simulink model "InvertedPendulum_DLQG_Simulink2020b"  (R2021b)
settings: Solver=ode4  StartTime=0.0  StopTime=SIM_TIME  FixedStep=STEP_SIZE  RelTol=1e-3
undefined symbols (not defined in the file): b, c, C_KF, F_KF, g, G_KF, I, K_opt, l, L_KF, m, M, N, theta0, theta_dot0, Ts, V2d, x0, x0_hat, x_dot0, x_ref0, yss
settings Model: Creator=roga  LastModifiedBy=roga
settings SolverCC: AlgebraicLoopSolver=TrustRegion
settings DataIOCC: ReturnWorkspaceOutputs=off
settings DebuggingCC: SFMachineParentedDataDiag=warning

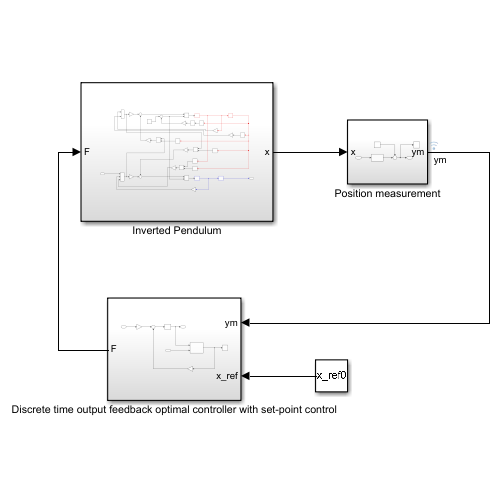
[thumbnail: Simulink's stored preview of the top-level diagram]
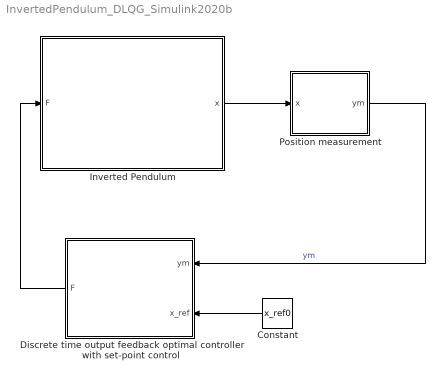
== system InvertedPendulum_DLQG_Simulink2020b ==
  Constant : Constant  Value=x_ref0  SampleTime=Ts
  Discrete time output feedback optimal controller with set-point control : Subsystem
  Inverted Pendulum : Subsystem
  Position measurement : Subsystem
  wires:
  Discrete time output feedback optimal controller with set-point control/1(F) -> Inverted Pendulum/1(F)
  Inverted Pendulum/1(x) -> Position measurement/1(x)
  Position measurement/1(ym) -> Discrete time output feedback optimal controller with set-point control/1(ym)  "ym"
  Constant/1 -> Discrete time output feedback optimal controller with set-point control/2(x_ref)

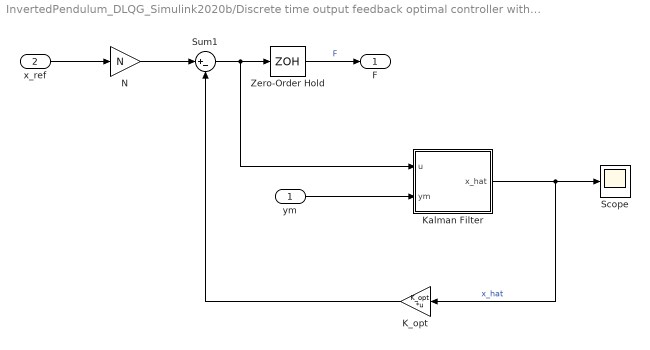
== system InvertedPendulum_DLQG_Simulink2020b/Discrete time output feedback optimal controller with set-point control ==
  ym : Inport
  x_ref : Inport  Port=2
  K_opt : Gain  Gain=K_opt  Multiplication=Matrix(K*u) (u vector)
  Kalman Filter : Subsystem
  N : Gain  Gain=N
  Scope : Scope
  Sum1 : Sum  Inputs=|+-
  Zero-Order Hold : ZeroOrderHold  SampleTime=Ts
  F : Outport
  wires:
  K_opt/1 -> Sum1/2
  Sum1/1 -> Kalman Filter/1(u), Zero-Order Hold/1
  Zero-Order Hold/1 -> F/1  "F"
  ym/1 -> Kalman Filter/2(ym)
  Kalman Filter/1(x_hat) -> Scope/1, K_opt/1  "x_hat"
  x_ref/1 -> N/1
  N/1 -> Sum1/1

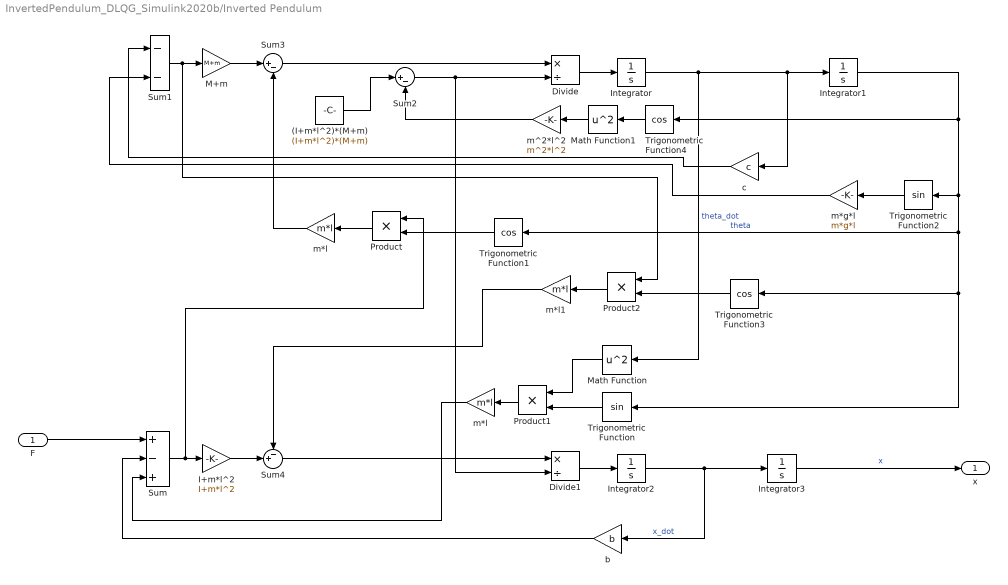
== system InvertedPendulum_DLQG_Simulink2020b/Inverted Pendulum ==
  F : Inport
  (I+m*l^2)*(M+m) : Constant  Value=(I+m*l^2)*(M+m)
  Divide : Product  Inputs=*/
  Divide1 : Product  Inputs=*/
  I+m*l^2 : Gain  Gain=I+m*l^2
  Integrator : Integrator  Priority=1  InitialCondition=theta_dot0  ContinuousStateAttributes='pendulum.angular.velocity'
  Integrator1 : Integrator  Priority=2  InitialCondition=theta0  UpperSaturationLimit=pi  LowerSaturationLimit=-pi  ContinuousStateAttributes='pendulum.angular.position'
  Integrator2 : Integrator  Priority=3  InitialCondition=x_dot0  ContinuousStateAttributes='trolley.horizontal.velocity'
  Integrator3 : Integrator  Priority=4  InitialCondition=x0  ContinuousStateAttributes='trolley.horizontal.position'
  M+m : Gain  Gain=M+m
  Math Function : Math  Operator=square  SaturateOnIntegerOverflow=on
  Math Function1 : Math  Operator=square  SaturateOnIntegerOverflow=on
  Product : Product
  Product1 : Product
  Product2 : Product
  Sum : Sum  Inputs=+-+
  Sum1 : Sum  Inputs=--
  Sum2 : Sum  Inputs=|+-
  Sum3 : Sum  Inputs=|+-
  Sum4 : Sum  Inputs=-+|
  Trigonometric Function : Trigonometry
  Trigonometric Function1 : Trigonometry  Operator=cos
  Trigonometric Function2 : Trigonometry
  Trigonometric Function3 : Trigonometry  Operator=cos
  Trigonometric Function4 : Trigonometry  Operator=cos
  b : Gain  Gain=b
  c : Gain  Gain=c
  m*g*l : Gain  Gain=m*g*l
  m*l : Gain  Gain=m*l
  "m*l " : Gain  Gain=m*l
  m*l1 : Gain  Gain=m*l
  m^2*l^2 : Gain  Gain=m^2*l^2
  x : Outport
  wires:
  Divide/1 -> Integrator/1
  m*l1/1 -> Sum4/1
  m*l/1 -> Sum3/2
  (I+m*l^2)*(M+m)/1 -> Sum2/1
  Math Function1/1 -> m^2*l^2/1
  Sum2/1 -> Divide1/2, Divide/2
  Divide1/1 -> Integrator2/1
  Product2/1 -> m*l1/1
  M+m/1 -> Sum3/1
  Sum4/1 -> Divide1/1
  I+m*l^2/1 -> Sum4/2
  Sum/1 -> Product/1, I+m*l^2/1
  Product1/1 -> "m*l "/1
  "m*l "/1 -> Sum/3
  Trigonometric Function2/1 -> m*g*l/1
  Integrator3/1 -> x/1  "x"
  Trigonometric Function1/1 -> Product/2
  Sum1/1 -> Product2/1, M+m/1
  Trigonometric Function3/1 -> Product2/2
  Integrator1/1 -> Trigonometric Function4/1, Trigonometric Function2/1, Trigonometric Function1/1, Trigonometric Function3/1, Trigonometric Function/1  "theta"
  m^2*l^2/1 -> Sum2/2
  Math Function/1 -> Product1/1
  m*g*l/1 -> Sum1/2
  Trigonometric Function/1 -> Product1/2
  b/1 -> Sum/2
  Integrator2/1 -> b/1, Integrator3/1  "x_dot"
  Integrator/1 -> Math Function/1, c/1, Integrator1/1  "theta_dot"
  c/1 -> Sum1/1
  Sum3/1 -> Divide/1
  Product/1 -> m*l/1
  Trigonometric Function4/1 -> Math Function1/1
  F/1 -> Sum/1

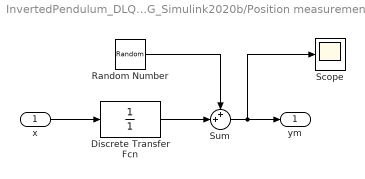
== system InvertedPendulum_DLQG_Simulink2020b/Position measurement ==
  x : Inport
  Discrete Transfer Fcn : DiscreteTransferFcn  Denominator=[1]  SampleTime=Ts
  Random Number : RandomNumber  Variance=V2d  Seed=[14973]  SampleTime=Ts
  Scope : Scope
  Sum : Sum  Inputs=++|
  ym : Outport
  wires:
  Sum/1 -> Scope/1, ym/1
  Random Number/1 -> Sum/1
  Discrete Transfer Fcn/1 -> Sum/2
  x/1 -> Discrete Transfer Fcn/1

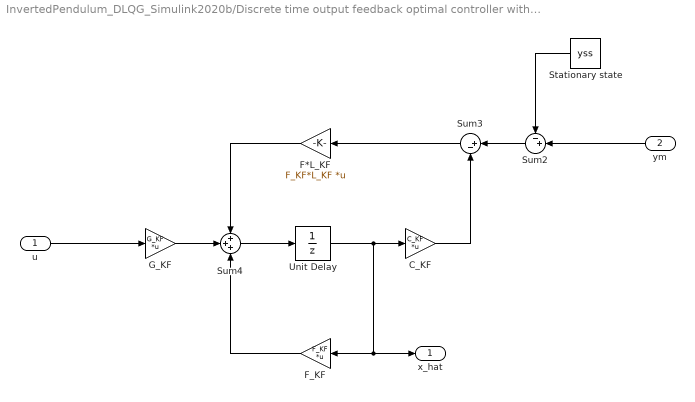
== system InvertedPendulum_DLQG_Simulink2020b/Discrete time output feedback optimal controller with set-point control/Kalman Filter ==
  u : Inport
  ym : Inport  Port=2
  C_KF : Gain  Gain=C_KF  Multiplication=Matrix(K*u) (u vector)
  F*L_KF : Gain  Gain=F_KF*L_KF  Multiplication=Matrix(K*u) (u vector)
  F_KF : Gain  Gain=F_KF  Multiplication=Matrix(K*u) (u vector)
  G_KF : Gain  Gain=G_KF  Multiplication=Matrix(K*u) (u vector)
  Stationary state : Constant  Value=yss
  Sum2 : Sum  Inputs=-+|
  Sum3 : Sum  Inputs=|+-
  Sum4 : Sum  Inputs=+++
  Unit Delay : UnitDelay  InitialCondition=x0_hat  SampleTime=Ts  HasFrameUpgradeWarning=on
  x_hat : Outport
  wires:
  F*L_KF/1 -> Sum4/1
  F_KF/1 -> Sum4/3
  G_KF/1 -> Sum4/2
  Unit Delay/1 -> x_hat/1, F_KF/1, C_KF/1
  Sum3/1 -> F*L_KF/1
  Stationary state/1 -> Sum2/1
  Sum4/1 -> Unit Delay/1
  Sum2/1 -> Sum3/1
  ym/1 -> Sum2/2
  u/1 -> G_KF/1
  C_KF/1 -> Sum3/2
